simulink model "bang"  (Simulink 7.9)
settings: Solver=ode45  StartTime=0.0  StopTime=abs(xdot/N)  RelTol=1e-6
values from neighbouring files (symbols this model uses):
  N = reshape(xx(n*nm+1:end),p,nm)    [Modelfollowingdesign.m]    (also in f_tos.m = 1; fig10_18.m = S\r; fig10_19.m = S\r; fig10_20.m = S\r)
undefined symbols (not defined in the file or in its folder): x, xdot
settings Model: Creator=abbas  LastModifiedBy=abbas
settings OptimizationCC: InlineInvariantSignals=on  InitFltsAndDblsToZero=on
settings DebuggingCC: SaveWithParameterizedLinksMsg=none  SignalResolutionControl=TryResolveAllWithWarning  SolverPrmCheckMsg=none  MultiTaskDSMMsg=warning  MultiTaskCondExecSysMsg=none  FcnCallInpInsideContextMsg=Use local settings  StrictBusMsg=None
settings RTWCC: IncludeERTFirstTime=on
settings GRTTargetCC: TargetFcnLib=ansi_tfl_tmw.mat  CombineOutputUpdateFcns=off  GRTInterface=on

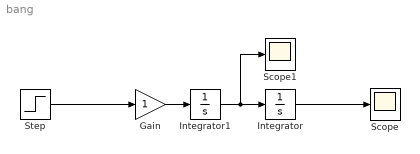
== system bang ==
  Gain : Gain
  Integrator : Integrator  InitialCondition=x
  Integrator1 : Integrator  InitialCondition=xdot
  Scope : Scope
      settings: SaveName=xbang
  Scope1 : Scope
      settings: SaveName=xdotbang
  Step : Step  Time=0  After=N  SampleTime=0
  wires:
  Integrator1/1 -> Integrator/1, Scope1/1
  Integrator/1 -> Scope/1
  Gain/1 -> Integrator1/1
  Step/1 -> Gain/1
